simulink subsystem "AC_bypass_pipe_accumulator"  (R2024b)
settings: Solver=VariableStepAuto  StartTime=0.0  StopTime=10.0  RelTol=1e-3
undefined symbols (not defined in the file): AC_bypass_line_port_inner_area, AC_bypass_pipe_length, Ambient_temp, Initial_temp, thermal_mass_per_length_bypass, wall_thickness
libraries: fl_lib x5, nesl_utility x2, SimscapeFluids_lib x1
settings Model: Creator=hc21562  LastModifiedBy=MW

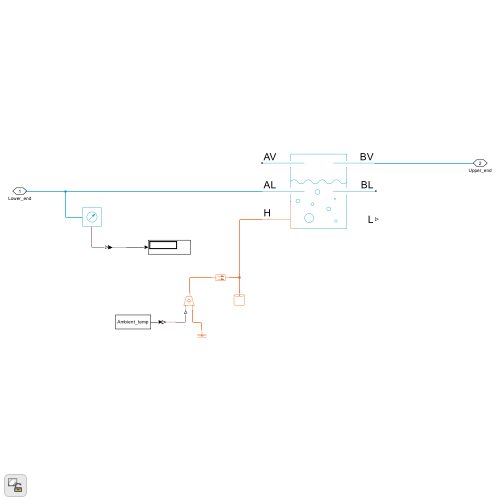
[thumbnail: Simulink's stored preview of the top-level diagram]
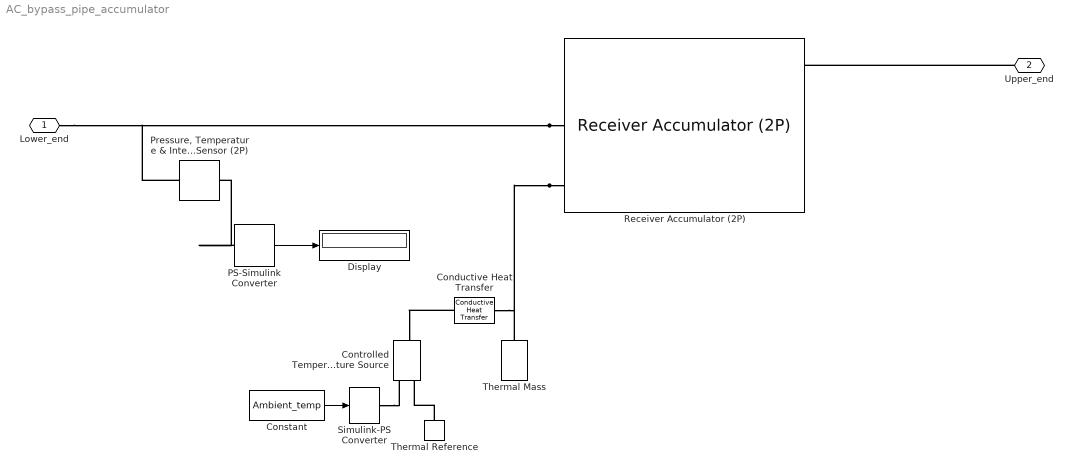
== system AC_bypass_pipe_accumulator ==
  Conductive Heat Transfer : fl_lib/Thermal/Thermal Elements/Conductive Heat Transfer  thermal_type=foundation.enum.ConstantVariableTabulated.Constant  wall_geometry=foundation.enum.ConductionWallGeometry.Cylindrical  area=hose_length m^2  thickness=0.01 m  d_in=AC_bypass_line_port_inner_area m  d_out=wall_thickness*2 + AC_bypass_line_port_inner_area m  L=AC_bypass_pipe_length m  th_cond_min=10 W/(K*m)  th_cond=pipe_thermal_conductivity W/(m*K)  th_cond_TLU=[413, 401, 392, 383, 371, 357, 342] W/(K*m)  temp_TLU=[200, 273, 400, 600, 800, 1000, 1200] K  T_specify=off  T_priority=None  T=0 K  T_nominal_specify=off  T_nominal_value=1  T_nominal_unit=K  Q_specify=off  Q_priority=None  Q=0 W  Q_nominal_specify=off  Q_nominal_value=1  Q_nominal_unit=W
  Constant : Constant  Value=Ambient_temp
  Controlled Temperature Source : fl_lib/Thermal/Thermal Sources/Controlled Temperature Source
  Display : Display
  PS-Simulink Converter : nesl_utility/PS-Simulink Converter  PhysicalDomain=network_engine_domain  SubClassName=ps_output  LeftPortType=input  RightPortType=output  PseudoPeriodic=off  Frequencies=[]  VectorFormat=inherit  Unit=inherit  AffineConversion=off
  "Pressure, Temperature & Internal Energy Sensor (2P)" : fl_lib/Two-Phase Fluid/Sensors/Pressure, Temperature & Internal Energy Sensor (2P)  reference=foundation.enum.MeasurementReference.absolute  pressure=false  pressure_spec=foundation.enum.PressureMeasementSpec.Absolute  temperature=false  internal_energy=true
      settings: InternalSimscapePortConfiguration="{\"Bottom\":[{\"id\":\"U\",\"label\":\"U\",\"type\":\"output\"}],\"Left\":[{\"id\":\"A\",\"label\":\"A\",\"type\":\"foundation.two_phase_fluid.two_phase_fluid\"}],\"Right\":[],\"Top\":[]}"
  Receiver Accumulator (2P) : SimscapeFluids_lib/Two-Phase Fluid/Tanks & Accumulators/Receiver Accumulator (2P)  volume=AC_bypass_pipe_length*AC_bypass_line_port_inner_area m^3  tank_area=AC_bypass_line_port_inner_area m^2  area_AV=AC_bypass_line_port_inner_area m^2  area_BV=AC_bypass_line_port_inner_area m^2  area_AL=AC_bypass_line_port_inner_area m^2  area_BL=AC_bypass_line_port_inner_area m^2  V_frac_liq_error=simscape.enum.assert.action.none  V_frac_liq_min=0.05  V_frac_liq_max=0.95  V_frac_smooth=0.05  p_crit_error=simscape.enum.assert.action.error  hc_vap=20 W/(K*m^2)  hc_liq=100 W/(K*m^2)  p_init=Initial_AC_tank_pressure bar  fraction_spec=fluids.two_phase_fluid.tanks_accumulators.enum.LiquidFractionSpec.Volume  M_frac_liq_init=0.5  V_frac_liq_init=0  saturated_init=false  energy_spec=fluids.two_phase_fluid.tanks_accumulators.enum.EnergySpec.Temperature  delta_T_sub_init=5 deltaK  delta_T_sup_init=5 deltaK  T_liq_init=Ambient_temp K  T_vap_init=Ambient_temp K  h_liq_init=400 kJ/kg  h_vap_init=2700 kJ/kg  u_liq_init=400 kJ/kg  u_vap_init=2700 kJ/kg  tau_vap_cond=0.1 s
      settings: InternalSimscapePortConfiguration="{\"Bottom\":[],\"Left\":[{\"id\":\"AV\",\"label\":\"AV\",\"type\":\"foundation.two_phase_fluid.two_phase_fluid\"},{\"id\":\"AL\",\"label\":\"AL\",\"type\":\"foundation.two_phase_fluid.two_phase_fluid\"},{\"id\":\"H\",\"label\":\"H\",\"type\":\"foundation.thermal.thermal\"}],\"Right\":[{\"id\":\"BV\",\"label\":\"BV\",\"type\":\"foundation.two_phase_fluid.two_phase_fluid\"},{\"id\":\"BL\",\"label\":\"BL\",\"type\":\"foundation.two_phase_fluid.two_phase_fluid\"},{\"id\":\"L\",\"label\":\"L\",\"type\":\"output\"}],\"Top\":[]}"
  Simulink-PS Converter : nesl_utility/Simulink-PS Converter  PhysicalDomain=network_engine_domain  SubClassName=ps_input  LeftPortType=input  RightPortType=output  PseudoPeriodic=off  Frequencies=[]  NoiseDistribution=none  NoiseParameters=[]  Unit=1  AffineConversion=off  FilteringAndDerivatives=zero  SimscapeFilterOrder=1  InputFilterTimeConstant=0.001  UdotUserProvided=1
  Thermal Mass : fl_lib/Thermal/Thermal Elements/Thermal Mass  mass_type=foundation.enum.constant_variable.constant  mass=thermal_mass_per_length_bypass*AC_bypass_pipe_length kg  sp_heat=steel_heat_capacity J/kg/K  mass_min=1e-6 kg  num_ports=foundation.enum.numPorts2.one  m_specify=off  m_priority=High  m=1 kg  m_nominal_specify=off  m_nominal_value=1  m_nominal_unit=kg  T_specify=on  T_priority=High  T=Initial_temp K  T_nominal_specify=off  T_nominal_value=1  T_nominal_unit=K  Q_specify=off  Q_priority=None  Q=0 W  Q_nominal_specify=off  Q_nominal_value=1  Q_nominal_unit=W
  Thermal Reference : fl_lib/Thermal/Thermal Elements/Thermal Reference
  Lower_end : PMIOPort  Side=Left
  Upper_end : PMIOPort  Port=2  Side=Right
  wires:
  Constant/1 -> Simulink-PS Converter/1
  PS-Simulink Converter/1 -> Display/1
  connections:
  Receiver Accumulator (2P)/LConn3 -- Thermal Mass/LConn1 -- Conductive Heat Transfer/RConn1
  Receiver Accumulator (2P)/LConn2 -- Lower_end/RConn1 -- "Pressure, Temperature & Internal Energy Sensor (2P)"/LConn1
  Thermal Reference/LConn1 -- Controlled Temperature Source/RConn2
  Simulink-PS Converter/RConn1 -- Controlled Temperature Source/RConn1
  Conductive Heat Transfer/LConn1 -- Controlled Temperature Source/LConn1
  Upper_end/RConn1 -- Receiver Accumulator (2P)/RConn1
  PS-Simulink Converter/LConn1 -- "Pressure, Temperature & Internal Energy Sensor (2P)"/RConn1
